simulink model "Cruise_control_System"  (R2022b)
settings: Solver=VariableStepAuto  StartTime=0.0  StopTime=inf  RelTol=1e-3
settings Model: Creator=Dell  LastModifiedBy=Dell

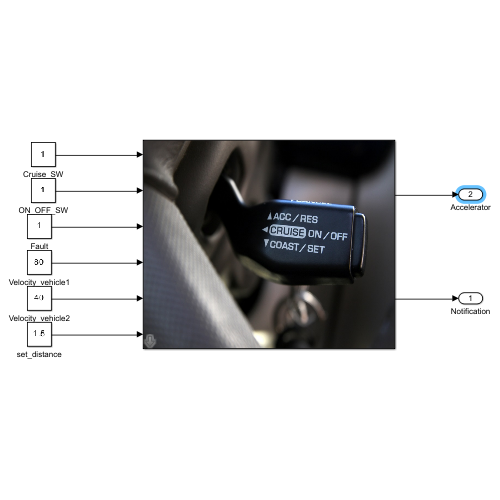
[thumbnail: Simulink's stored preview of the top-level diagram]
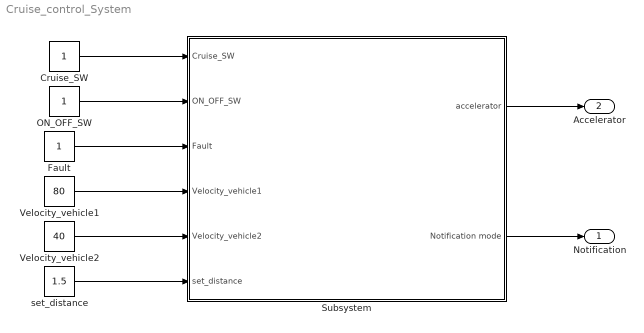
== system Cruise_control_System ==
  Cruise_SW : Constant
  Fault : Constant
  ON_OFF_SW : Constant
  Subsystem : Subsystem
      mask Display: image('cruise-control.jpg');
  Velocity_vehicle1 : Constant  Value=80
  Velocity_vehicle2 : Constant  Value=40
  set_distance : Constant  Value=1.5
  Notification : Outport
  Accelerator : Outport  Port=2
  wires:
  Cruise_SW/1 -> Subsystem/1(Cruise_SW)
  ON_OFF_SW/1 -> Subsystem/2(ON_OFF_SW)
  Fault/1 -> Subsystem/3(Fault)
  Velocity_vehicle1/1 -> Subsystem/4(Velocity_vehicle1)
  Velocity_vehicle2/1 -> Subsystem/5(Velocity_vehicle2)
  set_distance/1 -> Subsystem/6(set_distance)
  Subsystem/2(Notification mode) -> Notification/1
  Subsystem/1(accelerator) -> Accelerator/1

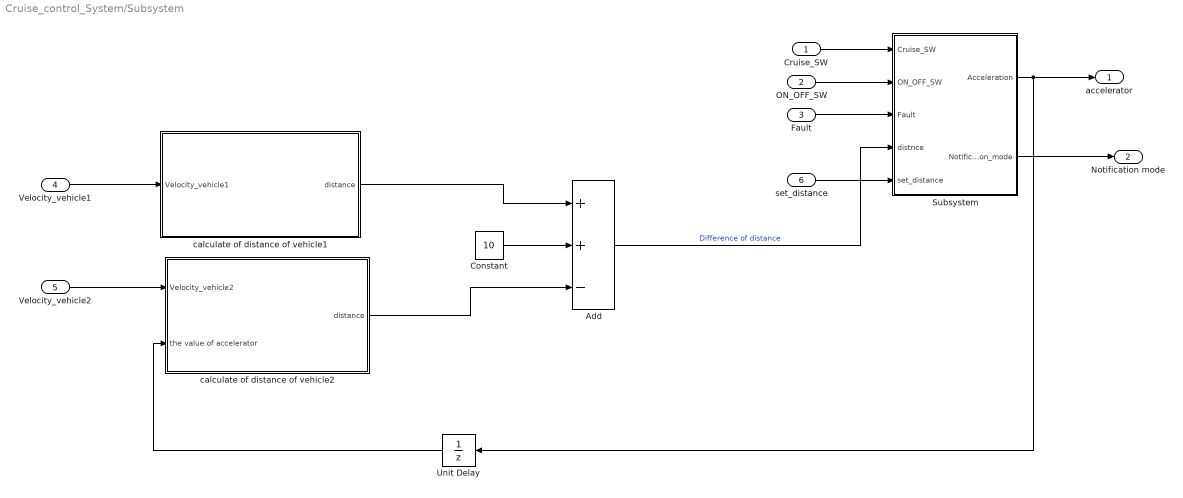
== system Cruise_control_System/Subsystem ==
  Cruise_SW : Inport
  ON_OFF_SW : Inport  Port=2
  Fault : Inport  Port=3
  Velocity_vehicle1 : Inport  Port=4
  Velocity_vehicle2 : Inport  Port=5
  set_distance : Inport  Port=6
  Add : Sum  Inputs=++-
  Constant : Constant  Value=10
  Subsystem : Subsystem
  Unit Delay : UnitDelay  InitialCondition=1  SampleTime=-1  HasFrameUpgradeWarning=on
  calculate of distance of vehicle1 : Subsystem
  calculate of distance of vehicle2 : Subsystem
  accelerator : Outport
  Notification mode : Outport  Port=2
  wires:
  Velocity_vehicle1/1 -> calculate of distance of vehicle1/1(Velocity_vehicle1)
  Velocity_vehicle2/1 -> calculate of distance of vehicle2/1(Velocity_vehicle2)
  calculate of distance of vehicle1/1(distance) -> Add/1
  calculate of distance of vehicle2/1(distance) -> Add/3
  Constant/1 -> Add/2
  Cruise_SW/1 -> Subsystem/1(Cruise_SW)
  ON_OFF_SW/1 -> Subsystem/2(ON_OFF_SW)
  Fault/1 -> Subsystem/3(Fault)
  Subsystem/1(Acceleration) -> Unit Delay/1, accelerator/1
  Subsystem/2(Notification_mode) -> Notification mode/1
  Unit Delay/1 -> calculate of distance of vehicle2/2(the value of accelerator)
  Add/1 -> Subsystem/4(distnce)  "Difference of distance"
  set_distance/1 -> Subsystem/5(set_distance)

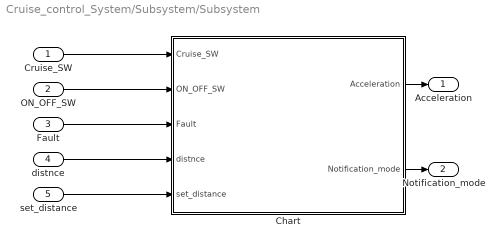
== system Cruise_control_System/Subsystem/Subsystem ==
  Cruise_SW : Inport
  ON_OFF_SW : Inport  Port=2
  Fault : Inport  Port=3
  distnce : Inport  Port=4
  set_distance : Inport  Port=5
  Chart : Stateflow chart  TreatAsAtomicUnit=on
      settings: PortSchema="{\"entries\":[{\"content\":{\"sides\":[{\"content\":{\"connectorIds\":[\"In2\",\"In3\",\"In4\",\"In1\",\"In5\"]},\"type\":\"ConnectorPlacement.EquallySpacedRectSide\",\"uuid\":\"4906a01a-7974-4c8e-ad8c-3bba2fae35ce\"},{\"content\":{\"connectorIds\":[\"Out1\",\"Out2\"],\"side\":\"RIGHT\"},\"type\":\"ConnectorPlacement.EquallySpacedRectSide\",\"uuid\":\"298045ce-a80b-4d65-b495-fb259af7d9cc\"},{\"content\":{\"connectorIds\":[],\"side\":\"TOP\"},\"type\":\"ConnectorPlacement.EquallySpacedRectSide\",\"uuid\":\"77697c85-b925-42a3-a98a-c483a43b3bb7\"},{\"content\":{\"connectorIds\":[],\"side\":\"BOTTOM\"},\"type\":\"ConnectorPlacement.EquallySpacedRectSide\",\"uuid\":\"9383277e-26f4-4ede-9f32-5cbb9c9713bc\"}]},\"type\":\"ConnectorPlacement.EquallySpacedConnector\",\"uuid\":\"2e41defc-b135-4677-951e-88f709dce39d\"}],\"packageUris\":[\"http://schema.mathworks.com/mf0/Connector/R2020b\"],\"version\":\"1.0\"}"
  Acceleration : Outport
  Notification_mode : Outport  Port=2
  wires:
  Cruise_SW/1 -> Chart/2(Cruise_SW)
  ON_OFF_SW/1 -> Chart/3(ON_OFF_SW)
  Fault/1 -> Chart/4(Fault)
  distnce/1 -> Chart/1(distnce)
  Chart/1(Acceleration) -> Acceleration/1
  Chart/2(Notification_mode) -> Notification_mode/1
  set_distance/1 -> Chart/5(set_distance)

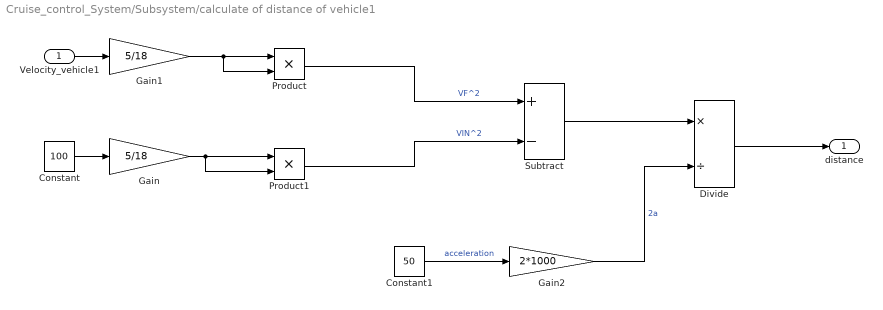
== system Cruise_control_System/Subsystem/calculate of distance of vehicle1 ==
  Velocity_vehicle1 : Inport
  Constant : Constant  Value=100
  Constant1 : Constant  Value=50
  Divide : Product  Inputs=*/
  Gain : Gain  Gain=5/18
  Gain1 : Gain  Gain=5/18
  Gain2 : Gain  Gain=2*1000
  Product : Product
  Product1 : Product
  Subtract : Sum  Inputs=+-
  distance : Outport
  wires:
  Velocity_vehicle1/1 -> Gain1/1
  Product/1 -> Subtract/1  "VF^2"
  Constant/1 -> Gain/1
  Gain/1 -> Product1/2, Product1/1
  Product1/1 -> Subtract/2  "VIN^2"
  Gain1/1 -> Product/2, Product/1
  Subtract/1 -> Divide/1
  Constant1/1 -> Gain2/1  "acceleration"
  Gain2/1 -> Divide/2  "2a"
  Divide/1 -> distance/1

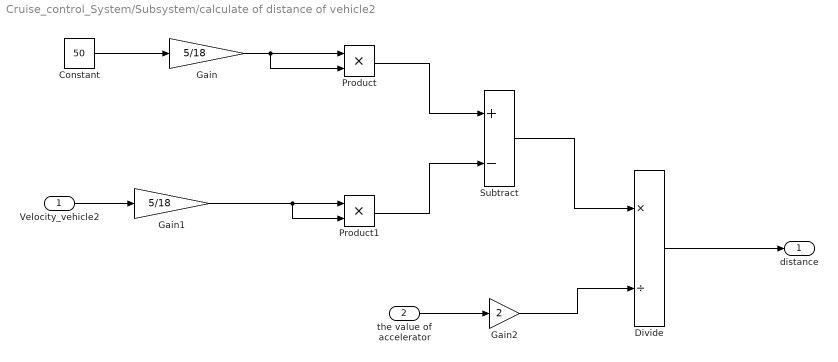
== system Cruise_control_System/Subsystem/calculate of distance of vehicle2 ==
  Velocity_vehicle2 : Inport
  the value of accelerator : Inport  Port=2
  Constant : Constant  Value=50
  Divide : Product  Inputs=*/
  Gain : Gain  Gain=5/18
  Gain1 : Gain  Gain=5/18
  Gain2 : Gain  Gain=2
  Product : Product
  Product1 : Product
  Subtract : Sum  Inputs=+-
  distance : Outport
  wires:
  Constant/1 -> Gain/1
  Velocity_vehicle2/1 -> Gain1/1
  Gain/1 -> Product/2, Product/1
  Gain1/1 -> Product1/2, Product1/1
  Product/1 -> Subtract/1
  Product1/1 -> Subtract/2
  the value of accelerator/1 -> Gain2/1
  Subtract/1 -> Divide/1
  Gain2/1 -> Divide/2
  Divide/1 -> distance/1

== stateflow chart Cruise_control_System/Subsystem/Subsystem/Chart ==
  state RegularSystem [parallel]
    settings: executionOrder=1
    state cruise_on
      (default) -> (junction 92)
      (junction 92) -> (junction 98)
      (junction 98) -> (junction 96) [order 1] : [distnce>15]
      (junction 98) -> (junction 90) [order 2]
      (junction 96) -> (junction 89) : {Notification_mode=System_mode.Accelerate; Acceleration = Acceleration +10;}
      (junction 89) -> (junction 90)
      (junction 90) -> (junction 86) [order 1] : [distnce < set_distance]
      (junction 90) -> (junction 87) [order 2]
      (junction 86) -> (junction 67) : {Notification_mode=System_mode.Stop;}
      (junction 67) -> (junction 87)
      (junction 87) -> (junction 69) [order 1] : [distnce<5]
      (junction 69) -> (junction 61) : {Notification_mode=System_mode.brake; Acceleration = Acceleration -20;}
      (junction 87) -> (junction 70) [order 2]
      (junction 61) -> (junction 70)
      (junction 70) -> (junction 66) [order 1] : [(distnce>5) && (distnce<10)]
      (junction 70) -> (junction 76) [order 2]
      (junction 66) -> (junction 71) : {Notification_mode=System_mode.Do_nothing; Acceleration = 1;}
      (junction 71) -> (junction 76)
      (junction 76) -> (junction 64) [order 1] : [distnce < 10]
      (junction 76) -> (junction 85) [order 2]
      (junction 64) -> (junction 62) : {Notification_mode=System_mode.Deaccelerate; Acceleration = Acceleration -10;}
      (junction 62) -> (junction 85)
      (junction 85) -> (junction 124)
    state cruise_off
      (default) -> (junction 104)
      (junction 104) -> (junction 106) [order 1] : [Fault==1]
      (junction 106) -> (junction 107) : {send(Local_fault_event,faultDetectionSystem);}
      (junction 104) -> (junction 108) [order 2] : {Notification_mode=System_mode.No_control_speed;}
      (junction 107) -> (junction 108)
      (junction 108) -> (junction 113)
    (default) -> cruise_on
    cruise_on -> cruise_off : [ (ON_OFF_SW==0) || (Cruise_SW==0) ||(Fault==1) ]
    cruise_off -> cruise_on : [ (ON_OFF_SW==1) && (Cruise_SW==1) &&(Fault==0) ]
  state faultDetectionSystem [parallel]
    settings: executionOrder=2
    state FaultMode
      Notification_mode=System_mode.Fault
    state withoutFault
      en:
    (default) -> withoutFault
    withoutFault -> FaultMode : Local_fault_event
  data: distnce input; Cruise_SW input; ON_OFF_SW input; Fault input; Acceleration output; Notification_mode output; set_distance input
  events: Local_fault_event local FUNCTION_CALL_EVENT
